simulink model "ForceControl_closed_loop"  (R2014a)
settings: Solver=ode23s  StartTime=0  StopTime=5  FixedStep=dt  MaxStep=50*dt  RelTol=1e-4
values from neighbouring files (symbols this model uses):
  alpha = Medium.alpha    [setConstants.m]
  amp_cl = eye(3)    [simulation_w_compensator.m]
  BmW = Misc.Bmag    [setConstants.m]
  ClosedLoop = 1    [simulation_w_compensator.m]
  h = 4.0693e-06    [forceControMatl.m]    (also in simulation_w_compensator.m)
  I = Dipole.inertia    [setConstants.m]
  kappa = -1.1700e-05    (= -1.17e-05)    [forceControMatl.m]    (also in simulation_w_compensator.m)
  Lx = xCoil.L    [setConstants.m]
  Ly = yCoil.L    [setConstants.m]
  m = Dipole.mass    [setConstants.m]
  M = Dipole.moment    [setConstants.m]
  Nx = xCoil.Turns    [setConstants.m]
  Ny = yCoil.Turns    [setConstants.m]
  Rx = xCoil.R+Rs    [setConstants.m]
  Ry = yCoil.R+Rs    [setConstants.m]
undefined symbols (not defined in the file or in its folder): Misc
libraries: cstblocks x2, dspsolvers x1
settings Model: Creator=Ron  LastModifiedBy=Ron
settings SolverCC: InitialStep=dt  MaxConsecutiveMinStep=5  ZeroCrossAlgorithm=Adaptive

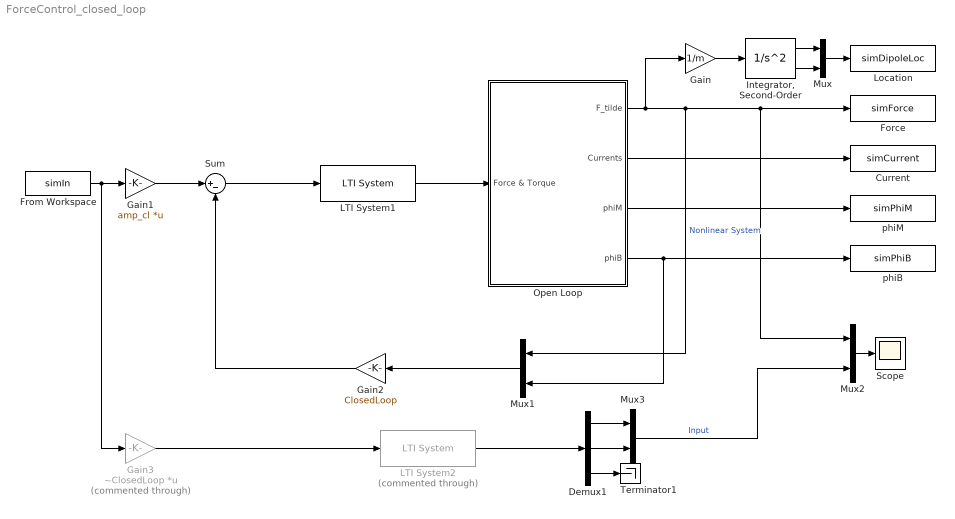
== system ForceControl_closed_loop ==
  Current : ToWorkspace  VariableName=simCurrent  SaveFormat=Timeseries  SampleTime=-1
  Demux1 : Demux  Outputs=3
  Force : ToWorkspace  VariableName=simForce  SaveFormat=Timeseries  SampleTime=-1
  From Workspace : FromWorkspace  VariableName=simIn  SampleTime=0
  Gain : Gain  Gain=1/m
  Gain1 : Gain  Gain=amp_cl  Multiplication=Matrix(K*u)
  Gain2 : Gain  Gain=ClosedLoop
  Gain3 : Gain  Commented=through  Gain=~ClosedLoop  Multiplication=Matrix(K*u)
  "Integrator, Second-Order" : SecondOrderIntegrator  ICX=initialValues.R0  ICDXDT=initialValues.V0
  LTI System1 : cstblocks/LTI System  sys=Ctf  IC=[0]
  LTI System2 : cstblocks/LTI System  Commented=through  sys=G_ol  IC=[0]
  Location : ToWorkspace  VariableName=simDipoleLoc  SaveFormat=Timeseries  SampleTime=-1
  Mux{,1..3} (4 alike) : Mux  Inputs=2
  Open Loop : Subsystem
  Scope : Scope
      settings: ShowLegends=on  YMin=-0.95  YMax=0
  Sum : Sum  Inputs=|+-
  Terminator1 : Terminator
  phiB : ToWorkspace  VariableName=simPhiB  SaveFormat=Timeseries  SampleTime=-1
  phiM : ToWorkspace  VariableName=simPhiM  SaveFormat=Timeseries  SampleTime=-1
  wires:
  Open Loop/1(F_tilde) -> Mux1/1, Mux2/1, Force/1, Gain/1  "Nonlinear System"
  Open Loop/2(Currents) -> Current/1
  "Integrator, Second-Order"/2 -> Mux/2
  Gain/1 -> "Integrator, Second-Order"/1
  Mux/1 -> Location/1
  "Integrator, Second-Order"/1 -> Mux/1
  Open Loop/3(phiM) -> phiM/1
  Open Loop/4(phiB) -> Mux1/2, phiB/1
  Sum/1 -> LTI System1/1
  From Workspace/1 -> Gain3/1, Gain1/1
  LTI System1/1 -> Open Loop/1(" Force & Torque")
  Gain1/1 -> Sum/1
  Mux1/1 -> Gain2/1
  Gain2/1 -> Sum/2
  Mux2/1 -> Scope/1
  Demux1/1 -> Mux3/1
  Demux1/2 -> Mux3/2
  Demux1/3 -> Terminator1/1
  LTI System2/1 -> Demux1/1
  Mux3/1 -> Mux2/2  "Input"
  Gain3/1 -> LTI System2/1

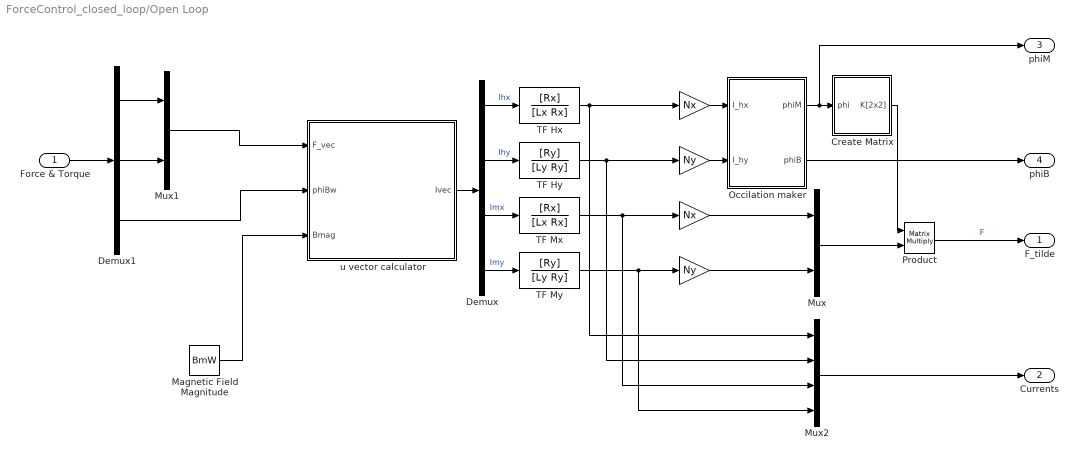
== system ForceControl_closed_loop/Open Loop ==
  " Force & Torque" : Inport
  "  " : Gain  Gain=Nx
  "   " : Gain  Gain=Nx
  "      " : Gain  Gain=Ny
  "            " : Gain  Gain=Ny
  Create Matrix : Subsystem
  Demux : Demux
  Demux1 : Demux  Outputs=3
  Magnetic Field Magnitude : Constant  Value=BmW
  Mux : Mux  Inputs=2
  Mux1 : Mux  Inputs=2
  Mux2 : Mux
  Occilation maker : Subsystem  TreatAsAtomicUnit=on
      mask Display:
      | disp('Solve\n Nonlinear\n Oscillation\n Equation')
      | % port_label('output', 1, 'phiM')
      | % port_label('input', 1, 'phiB')
      | % port_label('input', 2, 'Bmag')
  Product : Product  Multiplication=Matrix(*)
  TF Hx : TransferFcn  Numerator=[Rx]  Denominator=[Lx Rx]
  TF Hy : TransferFcn  Numerator=[Ry]  Denominator=[Ly Ry]
  TF Mx : TransferFcn  Numerator=[Rx]  Denominator=[Lx Rx]
  TF My : TransferFcn  Numerator=[Ry]  Denominator=[Ly Ry]
  u vector calculator : Subsystem
      mask Display:
      | disp('Calculate \n Input Variables ')
      | disp('\n\n\n By Input Force')
      | port_label('input',1,'Fvec')
      | port_label('input',2,'phiB')
      | port_label('input',3,'Bmag')
      | port_label('output',1,'Iw')
  F_tilde : Outport
  Currents : Outport  Port=2
  phiM : Outport  Port=3
  phiB : Outport  Port=4
  wires:
  TF Hy/1 -> "      "/1, Mux2/2
  TF Hx/1 -> Mux2/1, "  "/1
  Demux/2 -> TF Hy/1  "Ihy"
  Demux/4 -> TF My/1  "Imy"
  Demux/3 -> TF Mx/1  "Imx"
  Demux/1 -> TF Hx/1  "Ihx"
  Mux1/1 -> u vector calculator/1(F_vec)
  Magnetic Field Magnitude/1 -> u vector calculator/3(Bmag)
  Product/1 -> F_tilde/1  "F"
  Occilation maker/1(phiM) -> phiM/1, Create Matrix/1(phi)
  Demux1/3 -> u vector calculator/2(phiBw)
  Demux1/2 -> Mux1/2
  u vector calculator/1(Ivec) -> Demux/1
  Demux1/1 -> Mux1/1
  Create Matrix/1(K[2x2]) -> Product/1
  "      "/1 -> Occilation maker/2(I_hy)
  Mux/1 -> Product/2
  "            "/1 -> Mux/2
  TF My/1 -> "            "/1, Mux2/4
  "   "/1 -> Mux/1
  TF Mx/1 -> "   "/1, Mux2/3
  "  "/1 -> Occilation maker/1(I_hx)
  Mux2/1 -> Currents/1
  Occilation maker/2(phiB) -> phiB/1
  " Force & Torque"/1 -> Demux1/1

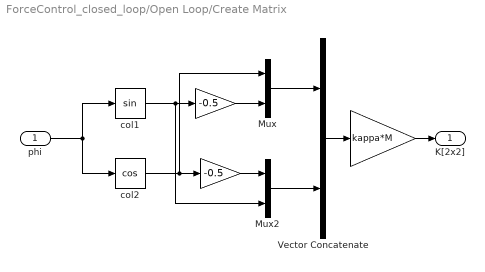
== system ForceControl_closed_loop/Open Loop/Create Matrix ==
  phi : Inport
  " " : Gain  Gain=-0.5
  "  " : Gain  Gain=-0.5
  "   " : Gain  Gain=kappa*M
  Mux : Mux  Inputs=2
  Mux2 : Mux  Inputs=2
  Vector Concatenate : Concatenate  Mode=Multidimensional array  ConcatenateDimension=2
  col1 : Trigonometry
  col2 : Trigonometry  Operator=cos
  K[2x2] : Outport
  wires:
  Mux2/1 -> Vector Concatenate/2
  " "/1 -> Mux/2
  col2/1 -> Mux/1, "  "/1
  phi/1 -> col2/1, col1/1
  col1/1 -> " "/1, Mux2/2
  Vector Concatenate/1 -> "   "/1
  "   "/1 -> K[2x2]/1
  Mux/1 -> Vector Concatenate/1
  "  "/1 -> Mux2/1

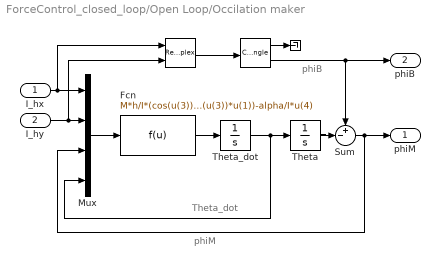
== system ForceControl_closed_loop/Open Loop/Occilation maker ==
  note: phiB
  note: Theta_dot
  note: phiM
  I_hx : Inport
  I_hy : Inport  Port=2
  " " : RealImagToComplex
  "  " : Terminator
  "   " : ComplexToMagnitudeAngle
  Fcn : Fcn  Expr=M*h/I*(cos(u(3))*u(2)-sin(u(3))*u(1))-alpha/I*u(4)
  Mux : Mux
  Sum : Sum  Inputs=+-|
  "Theta " : Integrator  ContinuousStateAttributes='alpha'
  Theta_dot : Integrator  ContinuousStateAttributes='alpha_dot'
  phiM : Outport
  phiB : Outport  Port=2
  wires:
  Theta_dot/1 -> Mux/4, "Theta "/1
  Fcn/1 -> Theta_dot/1
  Mux/1 -> Fcn/1
  I_hx/1 -> Mux/1, " "/1
  I_hy/1 -> " "/2, Mux/2
  " "/1 -> "   "/1
  "   "/2 -> phiB/1, Sum/1
  "Theta "/1 -> Sum/2
  Sum/1 -> Mux/3, phiM/1
  "   "/1 -> "  "/1

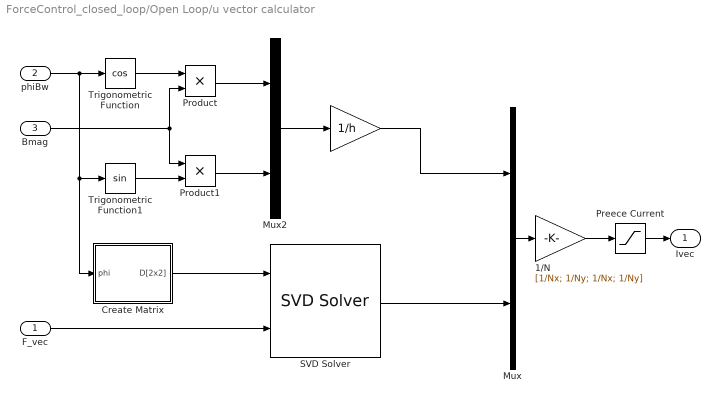
== system ForceControl_closed_loop/Open Loop/u vector calculator ==
  F_vec : Inport
  phiBw : Inport  Port=2
  Bmag : Inport  Port=3
  " " : Gain  Gain=1/h
  " 1/N" : Gain  Gain=[1/Nx; 1/Ny; 1/Nx; 1/Ny]
  Create Matrix : Subsystem
  Mux : Mux  Inputs=2
  Mux2 : Mux  Inputs=2
  Preece Current : Saturate  UpperLimit=Misc.maxCurr  LowerLimit=-Misc.maxCurr  ZeroCross=off
  Product : Product
  Product1 : Product
  SVD Solver : dspsolvers/SVD Solver  wanterr=off
  Trigonometric Function : Trigonometry  Operator=cos
  Trigonometric Function1 : Trigonometry
  Ivec : Outport
  wires:
  phiBw/1 -> Create Matrix/1(phi), Trigonometric Function1/1, Trigonometric Function/1
  Trigonometric Function/1 -> Product/1
  Trigonometric Function1/1 -> Product1/2
  Bmag/1 -> Product/2, Product1/1
  Product/1 -> Mux2/1
  Mux/1 -> " 1/N"/1
  Create Matrix/1(D[2x2]) -> SVD Solver/1
  F_vec/1 -> SVD Solver/2
  Mux2/1 -> " "/1
  Product1/1 -> Mux2/2
  Preece Current/1 -> Ivec/1
  " "/1 -> Mux/1
  SVD Solver/1 -> Mux/2
  " 1/N"/1 -> Preece Current/1

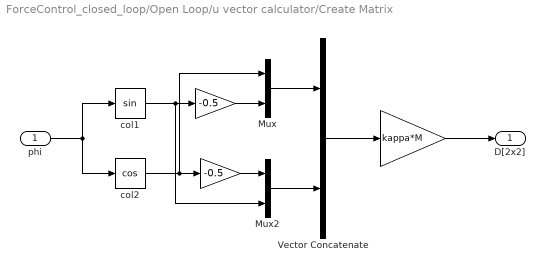
== system ForceControl_closed_loop/Open Loop/u vector calculator/Create Matrix ==
  phi : Inport
  " " : Gain  Gain=-0.5
  "  " : Gain  Gain=-0.5
  "   " : Gain  Gain=kappa*M
  Mux : Mux  Inputs=2
  Mux2 : Mux  Inputs=2
  Vector Concatenate : Concatenate  Mode=Multidimensional array  ConcatenateDimension=2
  col1 : Trigonometry
  col2 : Trigonometry  Operator=cos
  D[2x2] : Outport
  wires:
  Mux2/1 -> Vector Concatenate/2
  " "/1 -> Mux/2
  col2/1 -> Mux/1, "  "/1
  phi/1 -> col2/1, col1/1
  col1/1 -> " "/1, Mux2/2
  Vector Concatenate/1 -> "   "/1
  "   "/1 -> D[2x2]/1
  Mux/1 -> Vector Concatenate/1
  "  "/1 -> Mux2/1
